simulink model "SIL_model"  (R2020a)
settings: Solver=ode4  StartTime=0.0  StopTime=30  FixedStep=0.001  RelTol=1e-3
InitFcn:
  | Init_control;
values from neighbouring files (symbols this model uses):
  layer1 = double(results{1,1}.layer9)    [load_parameter.m]
  layer2 = double(results{1,1}.layer10)    [load_parameter.m]
  layer3 = double(results{1,1}.layer11)    [load_parameter.m]
  layer4 = double(results{1,1}.layer12)    [load_parameter.m]
  layer5 = double(results{1,1}.layer13)    [load_parameter.m]
  layer6 = double(results{1,1}.layer14)    [load_parameter.m]
  std = sqrt(max(a,0.01))    [load_parameter.m]
undefined symbols (not defined in the file or in its folder): DWORK0, DWORK1, DWORK10, DWORK11, DWORK12, DWORK13, DWORK14, DWORK15, DWORK2, DWORK3, DWORK4, DWORK5, DWORK6, DWORK7, DWORK8, DWORK9, earthRadius, KiPitchAttitude, KiRollAttitude, Kp_RP_ANGLE, MAX_CONTROL_ANGLE_RATE_Y, MAX_CONTROL_ANGLE_RP, ModelInit_RPM, ModelParam_envAltitude, ModelParam_GlobalNoiseGainSwitch, ModelParam_GPSLatLong, ModelParam_motorCr, ModelParam_motorJm, ModelParam_motorMinThr, ModelParam_motorT, ModelParam_motorWb, ModelParam_rotorCm, ModelParam_rotorCt, ModelParam_uavCCm, ModelParam_uavCd, ModelParam_uavDearo, ModelParam_uavJ, ModelParam_uavMass, ModelParam_uavR, ModelParam_uavType, Receive, Send
libraries: aerolibfltsims x4, simulink x2, shared6dof x1, aerolibanimutils x1
(part 1 of 2)
settings Model: SimulationMode=accelerator  Creator=dream  LastModifiedBy=NEW
settings DataIOCC: ReturnWorkspaceOutputs=off
settings DebuggingCC: BusObjectLabelMismatch=error  ArithmeticOperatorsInVariantConditions=warning
settings SFSimCC: SimUseLocalCustomCode=off  CustomCodeUndefinedFunction=UseInterfaceOnly
settings RTWCC: RTWUseLocalCustomCode=off
settings CodeAppCC: StateflowObjectComments=on

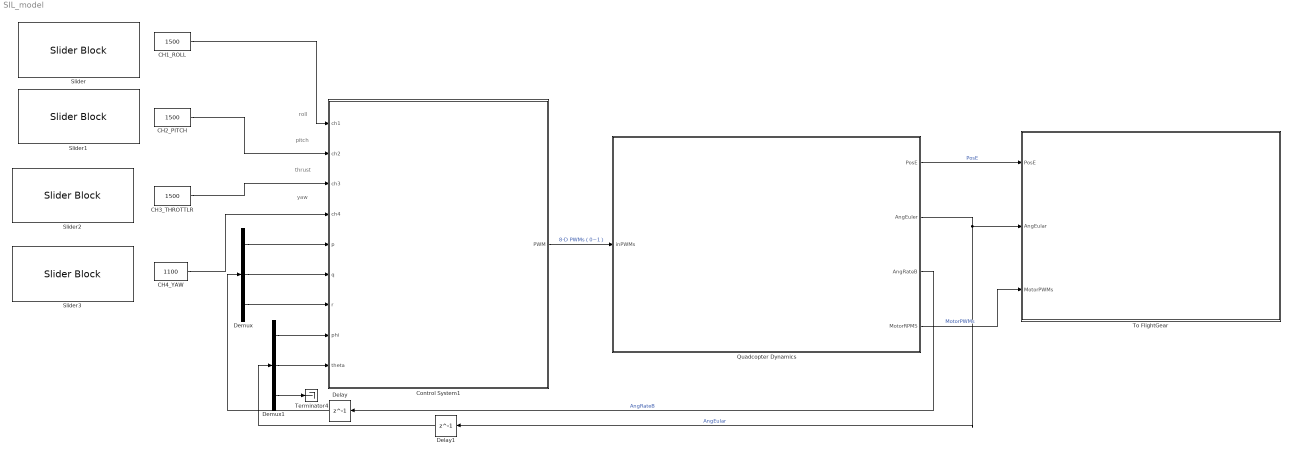
== system SIL_model ==
  note: roll
  note: pitch
  note: thrust
  note: yaw
  "     CH3_THROTTLR " : Constant  Value=1500  OutDataTypeStr=uint16
  "     CH4_YAW     " : Constant  Value=1100  OutDataTypeStr=uint16
  " CH2_PITCH " : Constant  Value=1500  OutDataTypeStr=uint16
  "CH1_ROLL   " : Constant  Value=1500  OutDataTypeStr=uint16
  Control System1 : Subsystem
      mask Display: image('icon\pixhawk.png');
  Delay : Delay  DelayLength=1  InitialCondition=0
  Delay1 : Delay  DelayLength=1  InitialCondition=0
  Demux : Demux  Outputs=3
  Demux1 : Demux  Outputs=3
  Quadcopter Dynamics : Subsystem
      mask Display: image('icon/F450.png');
  Slider : SliderBlock  ScaleMin=1100  ScaleMax=1900
  Slider1 : SliderBlock  ScaleMin=1100  ScaleMax=1900
  Slider2 : SliderBlock  ScaleMin=1500  ScaleMax=1680
  Slider3 : SliderBlock  ScaleMin=1100  ScaleMax=1900
  Terminator4 : Terminator
  To FlightGear : Subsystem
      mask Display: image('icon/FlightGear.png');
  wires:
  Quadcopter Dynamics/1(PosE) -> To FlightGear/1(PosE)  "PosE"
  Quadcopter Dynamics/2(AngEuler) -> To FlightGear/2(AngEular), Delay1/1  "AngEular"
  "CH1_ROLL   "/1 -> Control System1/1(ch1)
  "     CH4_YAW     "/1 -> Control System1/4(ch4)
  "     CH3_THROTTLR "/1 -> Control System1/3(ch3)
  Quadcopter Dynamics/3(AngRateB) -> Delay/1  "AngRateB"
  Demux/1 -> Control System1/5(p)
  Demux/2 -> Control System1/6(q)
  Demux/3 -> Control System1/7(r)
  Demux1/1 -> Control System1/8(phi)
  Demux1/2 -> Control System1/9(theta)
  Demux1/3 -> Terminator4/1
  " CH2_PITCH "/1 -> Control System1/2(ch2)
  Control System1/1(PWM) -> Quadcopter Dynamics/1(inPWMs)  "8-D PWMs（0~1）"
  Quadcopter Dynamics/4(MotorRPMS) -> To FlightGear/3(MotorPWMs)  "MotorPWMs"
  Delay/1 -> Demux/1
  Delay1/1 -> Demux1/1

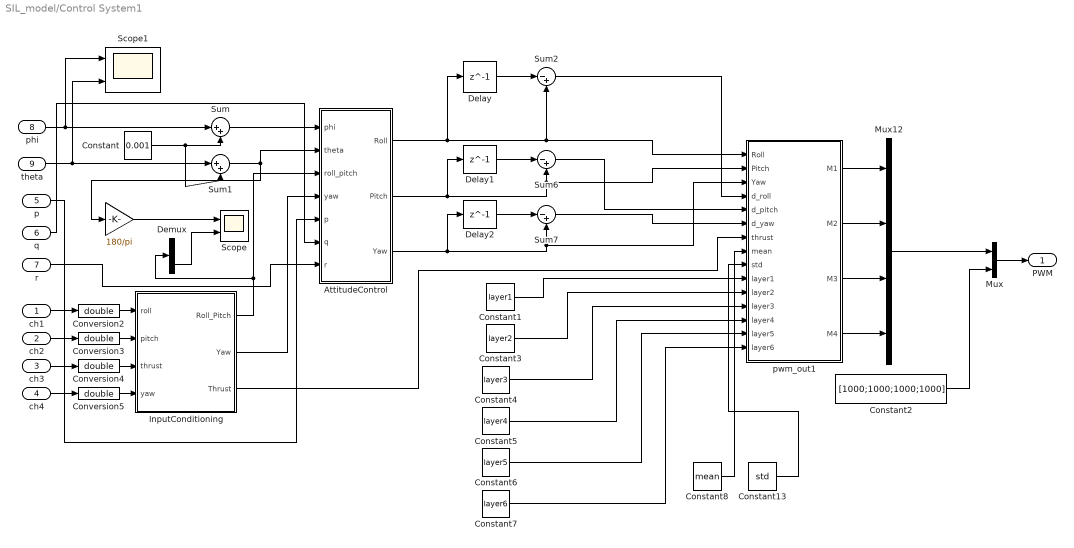
== system SIL_model/Control System1 ==
  ch1 : Inport  OutDataTypeStr=uint16  PortDimensions=1
  ch2 : Inport  Port=2  OutDataTypeStr=uint16  PortDimensions=1
  ch3 : Inport  Port=3  OutDataTypeStr=uint16  PortDimensions=1
  ch4 : Inport  Port=4  OutDataTypeStr=uint16  PortDimensions=1
  p : Inport  Port=5  PortDimensions=1
  q : Inport  Port=6  PortDimensions=1
  r : Inport  Port=7  PortDimensions=1
  phi : Inport  Port=8  PortDimensions=1
  theta : Inport  Port=9  PortDimensions=1
  " " : Gain  Gain=180/pi
  AttitudeControl : Subsystem
  Constant : Constant  Value=0.001
  Constant1 : Constant  Value=layer1
  Constant13 : Constant  Value=std
  Constant2 : Constant  Value=[1000;1000;1000;1000]
  Constant3 : Constant  Value=layer2
  Constant4 : Constant  Value=layer3
  Constant5 : Constant  Value=layer4
  Constant6 : Constant  Value=layer5
  Constant7 : Constant  Value=layer6
  Constant8 : Constant  Value=mean
  Conversion{2..5} (4 alike) : DataTypeConversion  OutDataTypeStr=double
  Delay : Delay  DelayLength=1  InitialCondition=0
  Delay1 : Delay  DelayLength=1  InitialCondition=0
  Delay2 : Delay  DelayLength=1  InitialCondition=0
  Demux : Demux  Outputs=2
  InputConditioning : Subsystem
  Mux : Mux  Inputs=2
  Mux12 : Mux
  Scope : Scope  NumInputPorts=2
  Scope1 : Scope  NumInputPorts=2
  Sum : Sum  Inputs=|++
  Sum1 : Sum  Inputs=|++
  Sum2 : Sum  Inputs=|-+
  Sum6 : Sum  Inputs=|-+
  Sum7 : Sum  Inputs=|-+
  pwm_out1 : MATLAB Function  TreatAsAtomicUnit=on
  PWM : Outport  PortDimensions=8  VectorParamsAs1DForOutWhenUnconnected=off
  wires:
  InputConditioning/3(Thrust) -> pwm_out1/7(thrust)
  AttitudeControl/2(Pitch) -> Delay1/1, Sum6/2, pwm_out1/2(Pitch)
  AttitudeControl/1(Roll) -> Delay/1, Sum2/2, pwm_out1/1(Roll)
  ch3/1 -> Conversion4/1
  pwm_out1/1(M1) -> Mux12/1
  pwm_out1/3(M3) -> Mux12/3
  pwm_out1/2(M2) -> Mux12/2
  r/1 -> AttitudeControl/7(r)
  AttitudeControl/3(Yaw) -> Delay2/1, Sum7/2, pwm_out1/3(Yaw)
  InputConditioning/1(Roll_Pitch) -> Demux/1, AttitudeControl/3(roll_pitch)
  q/1 -> AttitudeControl/6(q)
  theta/1 -> Scope1/2, Sum1/1
  InputConditioning/2(Yaw) -> AttitudeControl/4(yaw)
  p/1 -> AttitudeControl/5(p)
  ch4/1 -> Conversion5/1
  pwm_out1/4(M4) -> Mux12/4
  ch1/1 -> Conversion2/1
  ch2/1 -> Conversion3/1
  Conversion2/1 -> InputConditioning/1(roll)
  Conversion5/1 -> InputConditioning/4(yaw)
  Conversion4/1 -> InputConditioning/3(thrust)
  Conversion3/1 -> InputConditioning/2(pitch)
  " "/1 -> Scope/1
  Demux/2 -> Scope/2
  phi/1 -> Scope1/1, Sum/1
  Sum/1 -> AttitudeControl/1(phi)
  Sum1/1 -> " "/1, AttitudeControl/2(theta)
  Constant/1 -> Sum1/2, Sum/2
  Constant2/1 -> Mux/2
  Mux12/1 -> Mux/1
  Mux/1 -> PWM/1
  Sum2/1 -> pwm_out1/4(d_roll)
  Delay1/1 -> Sum6/1
  Sum6/1 -> pwm_out1/5(d_pitch)
  Delay2/1 -> Sum7/1
  Sum7/1 -> pwm_out1/6(d_yaw)
  Constant8/1 -> pwm_out1/8(mean)
  Constant13/1 -> pwm_out1/9(std)
  Constant1/1 -> pwm_out1/10(layer1)
  Constant3/1 -> pwm_out1/11(layer2)
  Constant4/1 -> pwm_out1/12(layer3)
  Constant5/1 -> pwm_out1/13(layer4)
  Constant6/1 -> pwm_out1/14(layer5)
  Constant7/1 -> pwm_out1/15(layer6)
  Delay/1 -> Sum2/1

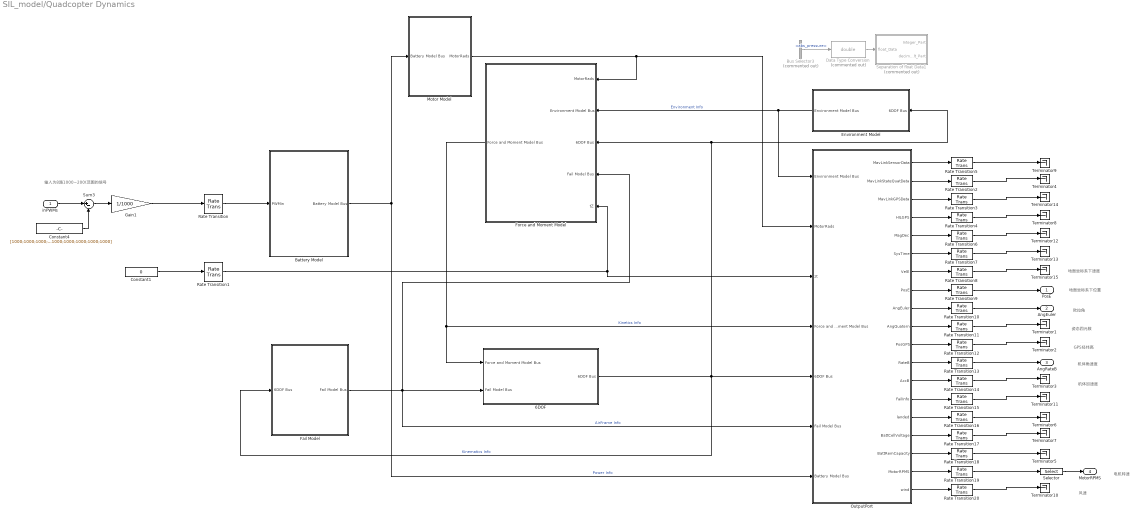
== system SIL_model/Quadcopter Dynamics ==
  note: 电机转速
  note: 风速
  note: 机体加速度
  note: 机体角速度
  note: GPS经纬高
  note: 姿态四元数
  note: 欧拉角
  note: 地面坐标系下位置
  note: 地面坐标系下速度
  note: 输入为8路1000~2000范围的信号
  inPWMs : Inport  PortDimensions=8
  6DOF : Subsystem
  Battery Model : Subsystem
      mask help: Simulink:masks:GenSFuncDesc_MD
      mask Help: eval('feval(''rtwprivate'',''rtwhelpview'',''rtw_sfcn_block'')');
  Bus Selector3 : BusSelector  Commented=on  OutputSignals=abs_pressure
  Constant1 : Constant  Value=0
  Constant4 : Constant  Value=[1000;1000;1000;1000;1000;1000;1000;1000]
  Data Type Conversion : DataTypeConversion  Commented=on  OutDataTypeStr=double
  Environment Model : Subsystem  mask{sfcnParam1=ModelParam_GPSLatLong, sfcnParam2=ModelParam_GlobalNoiseGainSwitch, sfcnParam3=ModelParam_envAltitude}
      mask prompts: sfcnParam1 "ModelParam_GPSLatLong:"; sfcnParam2 "ModelParam_GlobalNoiseGainSwitch:"; sfcnParam3 "ModelParam_envAltitude:"
      mask help: Simulink:masks:GenSFuncDesc_MD
      mask Help: eval('feval(''rtwprivate'',''rtwhelpview'',''rtw_sfcn_block'')');
  Fail Model : Subsystem  mask{sfcnParam1=ModelParam_uavJ, sfcnParam2=ModelParam_uavMass, sfcnParam3=ModelParam_uavR}
      mask prompts: sfcnParam1 "ModelParam_uavJ:"; sfcnParam2 "ModelParam_uavMass:"; sfcnParam3 "ModelParam_uavR:"
      mask help: Simulink:masks:GenSFuncDesc_MD
      mask Help: eval('feval(''rtwprivate'',''rtwhelpview'',''rtw_sfcn_block'')');
  Force and Moment Model : Subsystem  mask{sfcnParam1=ModelParam_motorJm, sfcnParam2=ModelParam_rotorCm, sfcnParam3=ModelParam_rotorCt, sfcnParam4=ModelParam_uavCCm, sfcnParam5=ModelParam_uavCd, sfcnParam6=ModelParam_uavDearo, sfcnParam7=ModelParam_uavR, sfcnParam8=ModelParam_uavType}
      mask prompts: sfcnParam1 "ModelParam_motorJm:"; sfcnParam2 "ModelParam_rotorCm:"; sfcnParam3 "ModelParam_rotorCt:"; sfcnParam4 "ModelParam_uavCCm:"; sfcnParam5 "ModelParam_uavCd:"; sfcnParam6 "ModelParam_uavDearo:"; sfcnParam7 "ModelParam_uavR:"; sfcnParam8 "ModelParam_uavType:"
      mask help: Simulink:masks:GenSFuncDesc_MD
      mask Help: eval('feval(''rtwprivate'',''rtwhelpview'',''rtw_sfcn_block'')');
  Gain1 : Gain  Gain=1/1000
  Motor Model : Subsystem  mask{sfcnParam1=ModelInit_RPM, sfcnParam2=ModelParam_motorCr, sfcnParam3=ModelParam_motorMinThr, sfcnParam4=ModelParam_motorT, sfcnParam5=ModelParam_motorWb}
      mask prompts: sfcnParam1 "ModelInit_RPM:"; sfcnParam2 "ModelParam_motorCr:"; sfcnParam3 "ModelParam_motorMinThr:"; sfcnParam4 "ModelParam_motorT:"; sfcnParam5 "ModelParam_motorWb:"
      mask help: Simulink:masks:GenSFuncDesc_MD
      mask Help: eval('feval(''rtwprivate'',''rtwhelpview'',''rtw_sfcn_block'')');
  OutputPort : Subsystem  mask{sfcnParam1=ModelParam_GPSLatLong, sfcnParam2=ModelParam_GlobalNoiseGainSwitch, sfcnParam3=ModelParam_envAltitude}
      mask prompts: sfcnParam1 "ModelParam_GPSLatLong:"; sfcnParam2 "ModelParam_GlobalNoiseGainSwitch:"; sfcnParam3 "ModelParam_envAltitude:"
      mask help: Simulink:masks:GenSFuncDesc_MD
      mask Help: eval('feval(''rtwprivate'',''rtwhelpview'',''rtw_sfcn_block'')');
  Rate Transition{,1..20} (21 alike) : RateTransition  OutPortSampleTime=ModelParam_BusSampleRate
  Selector : Selector  InputPortWidth=8  IndexOptions=Index vector (dialog)  Indices=[1 2 3 4]  OutputSizes=1
  Separation of float Data1 : Subsystem  Commented=on  mask{IntUint=1}
      mask prompts: IntUint "整数单位"
      mask help: 分离浮点数的整数和小数部分，这样在Labview MIT模块中可以稳定输出精度
  Sum3 : Sum  Inputs=|+-
  Terminator{1..15} (15 alike) : Terminator
  PosE : Outport  VectorParamsAs1DForOutWhenUnconnected=off
  AngEuler : Outport  Port=2  VectorParamsAs1DForOutWhenUnconnected=off
  AngRateB : Outport  Port=3  VectorParamsAs1DForOutWhenUnconnected=off
  MotorRPMS : Outport  Port=4  VectorParamsAs1DForOutWhenUnconnected=off
  wires:
  Selector/1 -> MotorRPMS/1
  Constant4/1 -> Sum3/2
  inPWMs/1 -> Sum3/1
  Constant1/1 -> Rate Transition1/1
  Sum3/1 -> Gain1/1
  Rate Transition5/1 -> Terminator9/1
  Rate Transition2/1 -> Terminator4/1
  Rate Transition3/1 -> Terminator14/1
  Rate Transition4/1 -> Terminator8/1
  Rate Transition6/1 -> Terminator12/1
  Rate Transition7/1 -> Terminator13/1
  Rate Transition8/1 -> Terminator15/1
  Rate Transition9/1 -> PosE/1
  Rate Transition10/1 -> AngEuler/1
  Rate Transition11/1 -> Terminator1/1
  Rate Transition12/1 -> Terminator2/1
  Rate Transition13/1 -> AngRateB/1
  Rate Transition14/1 -> Terminator3/1
  Rate Transition15/1 -> Terminator11/1
  Rate Transition16/1 -> Terminator6/1
  Rate Transition17/1 -> Terminator7/1
  Rate Transition18/1 -> Terminator5/1
  Rate Transition19/1 -> Selector/1
  Rate Transition20/1 -> Terminator10/1
  Gain1/1 -> Rate Transition/1
  OutputPort/2(MavLinkStateQuatData) -> Rate Transition2/1
  Motor Model/1(MotorRads) -> OutputPort/2(MotorRads), Force and Moment Model/1(MotorRads)
  OutputPort/15(landed) -> Rate Transition16/1
  OutputPort/3(MavLinkGPSData) -> Rate Transition3/1
  Bus Selector3/1 -> Data Type Conversion/1  "<abs_pressure>"
  Data Type Conversion/1 -> Separation of float Data1/1(float_Data)
  OutputPort/1(MavLinkSensorData) -> Rate Transition5/1
  OutputPort/14(FailInfo) -> Rate Transition15/1
  OutputPort/13(AccB) -> Rate Transition14/1
  OutputPort/12(RateB) -> Rate Transition13/1
  OutputPort/11(PosGPS) -> Rate Transition12/1
  OutputPort/10(AngQuatern) -> Rate Transition11/1
  OutputPort/9(AngEuler) -> Rate Transition10/1
  OutputPort/8(PosE) -> Rate Transition9/1
  OutputPort/7(VelE) -> Rate Transition8/1
  OutputPort/6(SysTime) -> Rate Transition7/1
  OutputPort/5(MagDec) -> Rate Transition6/1
  OutputPort/4(HILGPS) -> Rate Transition4/1
  Battery Model/1(Battery Model Bus) -> OutputPort/7(Battery Model Bus), Motor Model/1(Battery Model Bus)  "Power Info"
  Fail Model/1(Fail Model Bus) -> OutputPort/6(Fail Model Bus), Force and Moment Model/4(Fail Model Bus), 6DOF/2(Fail Model Bus)  "AirFrame Info"
  Force and Moment Model/1(Force and Moment Model Bus) -> OutputPort/4(Force and Moment Model Bus), 6DOF/1(Force and Moment Model Bus)  "Kinetics Info"
  6DOF/1(6DOF Bus) -> OutputPort/5(6DOF Bus), Fail Model/1(6DOF Bus), Environment Model/1(6DOF Bus), Force and Moment Model/3(6DOF Bus)  "Kinematics Info"
  Environment Model/1(Environment Model Bus) -> OutputPort/1(Environment Model Bus), Force and Moment Model/2(Environment Model Bus)  "Environment Info"
  OutputPort/16(BattCellVoltage) -> Rate Transition17/1
  OutputPort/17(BattRemCapacity) -> Rate Transition18/1
  OutputPort/19(wind) -> Rate Transition20/1
  OutputPort/18(MotorRPMS) -> Rate Transition19/1
  Rate Transition/1 -> Battery Model/1(PWMin)
  Rate Transition1/1 -> OutputPort/3(zt), Force and Moment Model/5("tZ ")

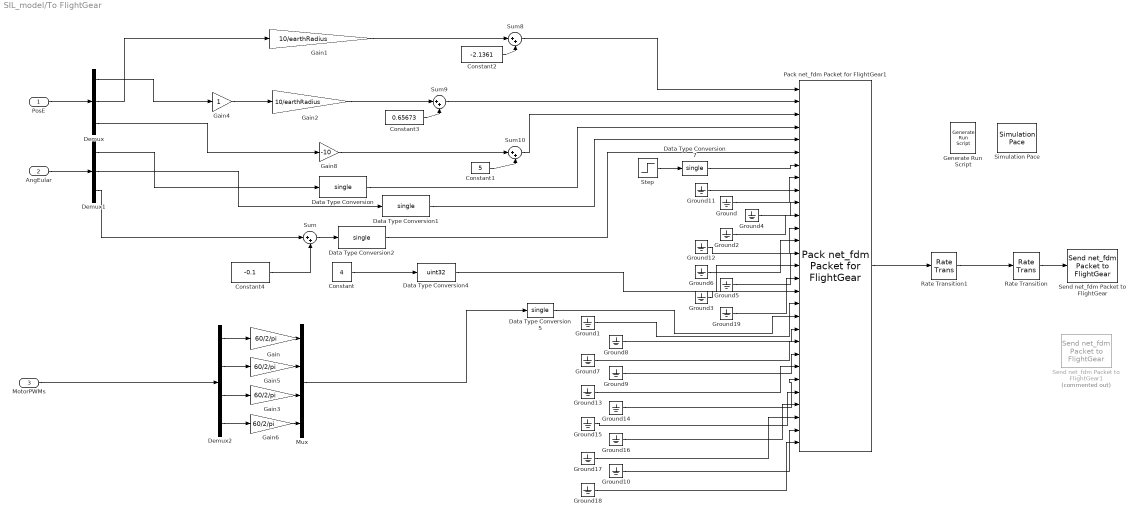
== system SIL_model/To FlightGear ==
  PosE : Inport
  AngEular : Inport  Port=2
  MotorPWMs : Inport  Port=3
  Constant : Constant  Value=4
  Constant1 : Constant  Value=5  VectorParams1D=off
  Constant2 : Constant  Value=-2.1361  VectorParams1D=off
  Constant3 : Constant  Value=0.65673  VectorParams1D=off
  Constant4 : Constant  Value=-0.1  VectorParams1D=off
  Data Type Conversion : DataTypeConversion  OutDataTypeStr=single  SaturateOnIntegerOverflow=on
  Data Type Conversion1 : DataTypeConversion  OutDataTypeStr=single  SaturateOnIntegerOverflow=on
  Data Type Conversion2 : DataTypeConversion  OutDataTypeStr=single  SaturateOnIntegerOverflow=on
  Data Type Conversion4 : DataTypeConversion  OutDataTypeStr=uint32
  Data Type Conversion5 : DataTypeConversion  OutDataTypeStr=single
  Data Type Conversion7 : DataTypeConversion  OutDataTypeStr=single
  Demux : Demux  Outputs=3
  Demux1 : Demux  Outputs=3
  Demux2 : Demux
  Gain{,3,5..6} (4 alike) : Gain  Gain=60/2/pi
  Gain1 : Gain  Gain=10/earthRadius
  Gain2 : Gain  Gain=10/earthRadius
  Gain4 : Gain
  Gain8 : Gain  Gain=-10
  Generate Run Script : aerolibfltsims/Generate Run Script  Architecture=Default  dataFlow=Send-Receive  GeometryModelName=Rotor4  AirportId=KSF0  RunwayId=10L  InitialAltitude=0  InitialHeading=0  OffsetDistance=0  OffsetAzimuth=0  InstallScenery=off  DisableShaders=off  OriginAddress=127.0.0.1  DestinationPort=5502  OriginPort=5505  LocalAddress=127.0.0.1  OutputFileName=runfg.bat  FlightGearBaseDirectory=C:\Program Files\FlightGear 2016.1.2
  Ground{,1..19} (20 alike) : Ground
  Mux : Mux
  Pack net_fdm Packet for FlightGear1 : aerolibfltsims/Pack net_fdm Packet for FlightGear  FlightGearVersion=v2016.1  ShowPositionAttitudeInputs=on  ShowVelocityAccelerationInputs=off  ShowControlSurfacePositionInputs=on  ShowEngineFuelInputs=on  ShowLandingGearInputs=off  ShowEnvironmentInputs=off  SampleTime=0.01  packetVersion=24
      settings: SourceProductBaseCode=AE
  Rate Transition : RateTransition
  Rate Transition1 : RateTransition
  Send net_fdm Packet to FlightGear : aerolibfltsims/Send net_fdm Packet to FlightGear  DestinationIpAddress=127.0.0.1  DestinationPort=5502  LocalIpPort=-1  varLen=off  SampleTime=0.005
      settings: SourceProductBaseCode=AE
  Send net_fdm Packet to FlightGear1 : aerolibfltsims/Send net_fdm Packet to FlightGear  Commented=on  DestinationIpAddress=192.168.199.46  DestinationPort=5502  LocalIpPort=-1  varLen=off  SampleTime=0.01
      settings: SourceProductBaseCode=AE
  Simulation Pace : aerolibanimutils/Simulation Pace  SimulationPace=1  SleepMode=MATLAB Thread  OutputPaceError=off  SampleTime=-1
      settings: AttributesFormatString=%<SimulationPace> sec/sec
  Step : Step  Time=5  SampleTime=0
  Sum{,8..10} (4 alike) : Sum  Inputs=|++
  wires:
  Rate Transition/1 -> Send net_fdm Packet to FlightGear/1
  Demux/1 -> Gain4/1
  Demux/2 -> Gain1/1
  Demux/3 -> Gain8/1
  Constant4/1 -> Sum/2
  Sum/1 -> Data Type Conversion2/1
  Gain1/1 -> Sum8/1
  Constant2/1 -> Sum8/2
  Gain2/1 -> Sum9/1
  Constant3/1 -> Sum9/2
  Constant1/1 -> Sum10/2
  Gain8/1 -> Sum10/1
  Pack net_fdm Packet for FlightGear1/1 -> Rate Transition1/1
  Demux1/2 -> Data Type Conversion1/1
  Demux1/3 -> Sum/1
  Data Type Conversion7/1 -> Pack net_fdm Packet for FlightGear1/7
  Ground8/1 -> Pack net_fdm Packet for FlightGear1/20
  Ground/1 -> Pack net_fdm Packet for FlightGear1/9
  Ground7/1 -> Pack net_fdm Packet for FlightGear1/21
  Ground9/1 -> Pack net_fdm Packet for FlightGear1/22
  Ground13/1 -> Pack net_fdm Packet for FlightGear1/23
  Ground14/1 -> Pack net_fdm Packet for FlightGear1/24
  Ground15/1 -> Pack net_fdm Packet for FlightGear1/25
  Ground16/1 -> Pack net_fdm Packet for FlightGear1/26
  Ground17/1 -> Pack net_fdm Packet for FlightGear1/27
  Ground10/1 -> Pack net_fdm Packet for FlightGear1/28
  Ground18/1 -> Pack net_fdm Packet for FlightGear1/29
  Step/1 -> Data Type Conversion7/1
  Data Type Conversion4/1 -> Pack net_fdm Packet for FlightGear1/17
  Ground1/1 -> Pack net_fdm Packet for FlightGear1/18
  Ground3/1 -> Pack net_fdm Packet for FlightGear1/15
  Ground5/1 -> Pack net_fdm Packet for FlightGear1/14
  Ground6/1 -> Pack net_fdm Packet for FlightGear1/13
  Ground4/1 -> Pack net_fdm Packet for FlightGear1/10
  Ground11/1 -> Pack net_fdm Packet for FlightGear1/8
  Data Type Conversion2/1 -> Pack net_fdm Packet for FlightGear1/6
  Data Type Conversion1/1 -> Pack net_fdm Packet for FlightGear1/5
  Data Type Conversion/1 -> Pack net_fdm Packet for FlightGear1/4
  Sum8/1 -> Pack net_fdm Packet for FlightGear1/1
  Sum9/1 -> Pack net_fdm Packet for FlightGear1/2
  Sum10/1 -> Pack net_fdm Packet for FlightGear1/3
  Constant/1 -> Data Type Conversion4/1
  Data Type Conversion5/1 -> Pack net_fdm Packet for FlightGear1/19
  Ground2/1 -> Pack net_fdm Packet for FlightGear1/11
  Ground12/1 -> Pack net_fdm Packet for FlightGear1/12
  Ground19/1 -> Pack net_fdm Packet for FlightGear1/16
  Gain4/1 -> Gain2/1
  AngEular/1 -> Demux1/1
  PosE/1 -> Demux/1
  MotorPWMs/1 -> Demux2/1
  Mux/1 -> Data Type Conversion5/1
  Demux2/1 -> Gain/1
  Demux2/3 -> Gain3/1
  Gain/1 -> Mux/1
  Gain3/1 -> Mux/3
  Demux2/2 -> Gain5/1
  Gain5/1 -> Mux/2
  Demux2/4 -> Gain6/1
  Gain6/1 -> Mux/4
  Demux1/1 -> Data Type Conversion/1
  Rate Transition1/1 -> Rate Transition/1

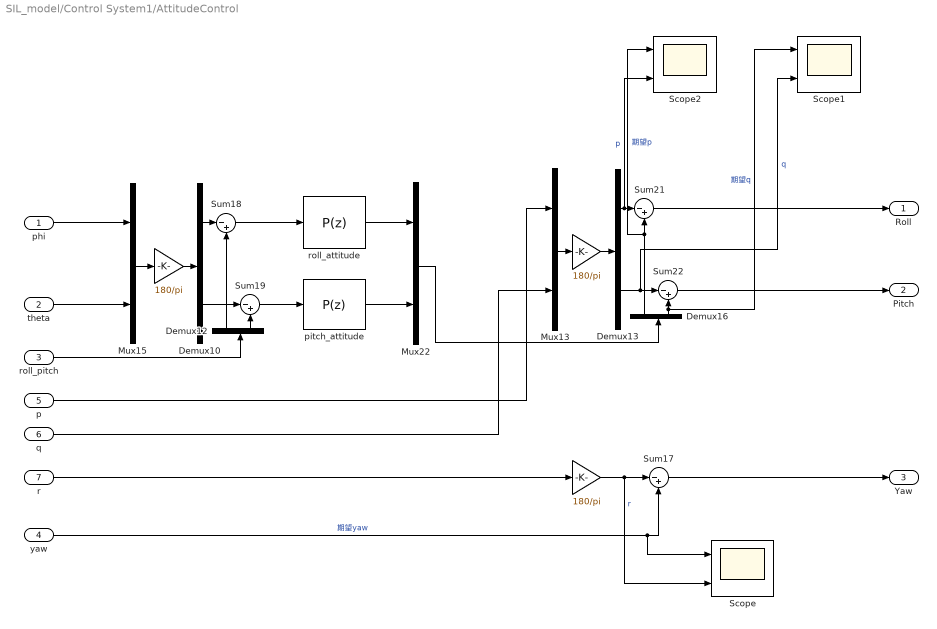
== system SIL_model/Control System1/AttitudeControl ==
  phi : Inport
  theta : Inport  Port=2
  roll_pitch : Inport  Port=3
  yaw : Inport  Port=4
  p : Inport  Port=5
  q : Inport  Port=6
  r : Inport  Port=7
  " " : Gain  Gain=180/pi
  "  " : Gain  Gain=180/pi
  "          " : Gain  Gain=180/pi
  Demux{10,12..13,16} (4 alike) : Demux  Outputs=2
  Mux13 : Mux  Inputs=2
  Mux15 : Mux  Inputs=2
  Mux22 : Mux  Inputs=2
  Scope : Scope  NumInputPorts=2
  Scope1 : Scope  NumInputPorts=2
  Scope2 : Scope  NumInputPorts=2
  Sum{17..19,21..22} (5 alike) : Sum  Inputs=|-+
  pitch_attitude : simulink/Continuous/PID Controller  Controller=P  Form=Parallel  TimeDomain=Discrete-time  UseExternalTs=off  SampleTime=-1  IntegratorMethod=Forward Euler  FilterMethod=Forward Euler  ControllerParametersSource=internal  P=Kp_RP_ANGLE  I=KiPitchAttitude  D=0.01  UseFilter=on  N=100  TunerSelectOption=Transfer Function Based (PID Tuner App)  InitialConditionSource=internal  InitialConditionForIntegrator=0  InitialConditionForFilter=0  DifferentiatorICPrevScaledInput=0  ExternalReset=none  TrackingMode=off  Kt=1  LimitOutput=on  UpperSaturationLimit=180  LowerSaturationLimit=-180  LinearizeAsGain=on  AntiWindupMode=back-calculation  Kb=1  POutMin=[]  POutMax=[]  IOutMin=[]  IOutMax=[]  DOutMin=[]  DOutMax=[]  NOutMin=[]  NOutMax=[]  SumOutMin=[]  SumOutMax=[]  SaturationOutMin=[]  SaturationOutMax=[]  PParamMin=[]  PParamMax=[]  IParamMin=[]  IParamMax=[]  DParamMin=[]  DParamMax=[]  NParamMin=[]  NParamMax=[]  KbParamMin=[]  KbParamMax=[]  KtParamMin=[]  KtParamMax=[]  KbOutMin=[]  KbOutMax=[]  KtOutMin=[]  KtOutMax=[]  IntegratorOutMin=[]  IntegratorOutMax=[]  FilterOutMin=[]  FilterOutMax=[]  SumI1OutMin=[]  SumI1OutMax=[]  SumI2OutMin=[]  SumI2OutMax=[]  SumI3OutMin=[]  SumI3OutMax=[]  SumI4OutMin=[]  SumI4OutMax=[]  SumDOutMin=[]  SumDOutMax=[]  DifferentiatorOutMin=[]  DifferentiatorOutMax=[]  FilterDiffOutCoefMin=[]  FilterDiffOutCoefMax=[]  ReciprocalOutMin=[]  ReciprocalOutMax=[]  SumDenOutMin=[]  SumDenOutMax=[]  SumNumOutMin=[]  SumNumOutMax=[]  DivideOutMin=[]  DivideOutMax=[]  UdiffTsProdOutMin=[]  UdiffTsProdOutMax=[]  NTsProdOutMin=[]  NTsProdOutMax=[]  UintegralTsProdOutMin=[]  UintegralTsProdOutMax=[]  UngainTsProdOutMin=[]  UngainTsProdOutMax=[]  IntegratorContinuousStateAttributes=''  IntegratorStateMustResolveToSignalObject=off  IntegratorRTWStateStorageClass=Auto  FilterContinuousStateAttributes=''  FilterStateMustResolveToSignalObject=off  FilterRTWStateStorageClass=Auto  ParallelPVariant=InternalParameters  IdealPVariant=Disabled  IVariant=Disabled  DVariant=Disabled  IntegratorVariant=Disabled  SatVariant=Enabled  AWVariant=Disabled  PCopyVariant=Disabled  TRVariant=Disabled  FdbkBlocksVariant=Forward  IdealPFdbkVariant=Disabled  SatFdbkVariant=Disabled  DerivativeFilterVariant=Disabled  NVariant=Disabled  NCopyVariant=Disabled_SignalSpec  FilterICVariant=Disabled  IntegratorICVariant=Disabled  ExternalResetVariant=Disabled  TRSumVariant=Passthrough  SumFdbkVariant=Disabled  SumVariant=Passthrough_P  TsampFilterVariant=InternalTs  TsampNgainVariant=Passthrough  TsampIntegralVariant=Disabled_SignalSpec
  roll_attitude : simulink/Continuous/PID Controller  Controller=P  Form=Parallel  TimeDomain=Discrete-time  UseExternalTs=off  SampleTime=-1  IntegratorMethod=Forward Euler  FilterMethod=Forward Euler  ControllerParametersSource=internal  P=Kp_RP_ANGLE  I=KiRollAttitude  D=0.01  UseFilter=on  N=100  TunerSelectOption=Transfer Function Based (PID Tuner App)  InitialConditionSource=internal  InitialConditionForIntegrator=0  InitialConditionForFilter=0  DifferentiatorICPrevScaledInput=0  ExternalReset=none  TrackingMode=off  Kt=1  LimitOutput=on  UpperSaturationLimit=180  LowerSaturationLimit=-180  LinearizeAsGain=on  AntiWindupMode=back-calculation  Kb=1  POutMin=[]  POutMax=[]  IOutMin=[]  IOutMax=[]  DOutMin=[]  DOutMax=[]  NOutMin=[]  NOutMax=[]  SumOutMin=[]  SumOutMax=[]  SaturationOutMin=[]  SaturationOutMax=[]  PParamMin=[]  PParamMax=[]  IParamMin=[]  IParamMax=[]  DParamMin=[]  DParamMax=[]  NParamMin=[]  NParamMax=[]  KbParamMin=[]  KbParamMax=[]  KtParamMin=[]  KtParamMax=[]  KbOutMin=[]  KbOutMax=[]  KtOutMin=[]  KtOutMax=[]  IntegratorOutMin=[]  IntegratorOutMax=[]  FilterOutMin=[]  FilterOutMax=[]  SumI1OutMin=[]  SumI1OutMax=[]  SumI2OutMin=[]  SumI2OutMax=[]  SumI3OutMin=[]  SumI3OutMax=[]  SumI4OutMin=[]  SumI4OutMax=[]  SumDOutMin=[]  SumDOutMax=[]  DifferentiatorOutMin=[]  DifferentiatorOutMax=[]  FilterDiffOutCoefMin=[]  FilterDiffOutCoefMax=[]  ReciprocalOutMin=[]  ReciprocalOutMax=[]  SumDenOutMin=[]  SumDenOutMax=[]  SumNumOutMin=[]  SumNumOutMax=[]  DivideOutMin=[]  DivideOutMax=[]  UdiffTsProdOutMin=[]  UdiffTsProdOutMax=[]  NTsProdOutMin=[]  NTsProdOutMax=[]  UintegralTsProdOutMin=[]  UintegralTsProdOutMax=[]  UngainTsProdOutMin=[]  UngainTsProdOutMax=[]  IntegratorContinuousStateAttributes=''  IntegratorStateMustResolveToSignalObject=off  IntegratorRTWStateStorageClass=Auto  FilterContinuousStateAttributes=''  FilterStateMustResolveToSignalObject=off  FilterRTWStateStorageClass=Auto  ParallelPVariant=InternalParameters  IdealPVariant=Disabled  IVariant=Disabled  DVariant=Disabled  IntegratorVariant=Disabled  SatVariant=Enabled  AWVariant=Disabled  PCopyVariant=Disabled  TRVariant=Disabled  FdbkBlocksVariant=Forward  IdealPFdbkVariant=Disabled  SatFdbkVariant=Disabled  DerivativeFilterVariant=Disabled  NVariant=Disabled  NCopyVariant=Disabled_SignalSpec  FilterICVariant=Disabled  IntegratorICVariant=Disabled  ExternalResetVariant=Disabled  TRSumVariant=Passthrough  SumFdbkVariant=Disabled  SumVariant=Passthrough_P  TsampFilterVariant=InternalTs  TsampNgainVariant=Passthrough  TsampIntegralVariant=Disabled_SignalSpec
  Roll : Outport  VectorParamsAs1DForOutWhenUnconnected=off
  Pitch : Outport  Port=2  VectorParamsAs1DForOutWhenUnconnected=off
  Yaw : Outport  Port=3  VectorParamsAs1DForOutWhenUnconnected=off
  wires:
  r/1 -> "          "/1
  q/1 -> Mux13/2
  Mux22/1 -> Demux16/1
  Sum17/1 -> Yaw/1
  phi/1 -> Mux15/1
  Mux15/1 -> " "/1
  theta/1 -> Mux15/2
  "          "/1 -> Scope/2, Sum17/1  "r"
  Sum19/1 -> pitch_attitude/1
  pitch_attitude/1 -> Mux22/2
  roll_attitude/1 -> Mux22/1
  Demux16/1 -> Scope2/1, Sum21/2  "期望p"
  yaw/1 -> Scope/1, Sum17/2  "期望yaw"
  roll_pitch/1 -> Demux12/1
  Demux16/2 -> Scope1/1, Sum22/2  "期望q"
  Demux12/1 -> Sum18/2
  Demux12/2 -> Sum19/2
  p/1 -> Mux13/1
  Demux10/1 -> Sum18/1
  Demux10/2 -> Sum19/1
  " "/1 -> Demux10/1
  Sum18/1 -> roll_attitude/1
  Sum22/1 -> Pitch/1
  Mux13/1 -> "  "/1
  Demux13/1 -> Scope2/2, Sum21/1  "p"
  Demux13/2 -> Scope1/2, Sum22/1  "q"
  "  "/1 -> Demux13/1
  Sum21/1 -> Roll/1

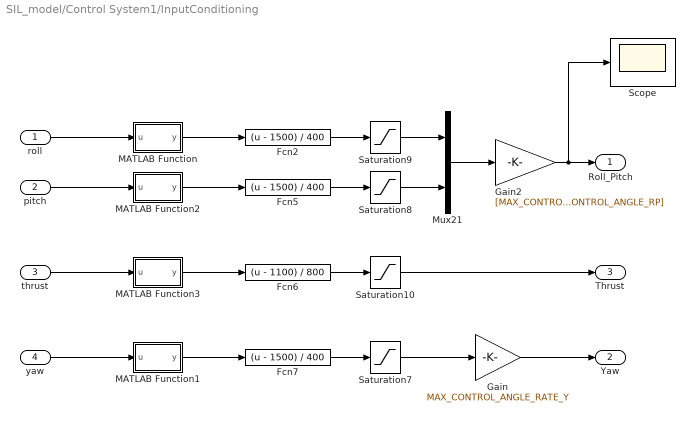
== system SIL_model/Control System1/InputConditioning ==
  roll : Inport
  pitch : Inport  Port=2
  thrust : Inport  Port=3
  yaw : Inport  Port=4
  Fcn2 : Fcn  Expr=(u - 1500) / 400
  Fcn5 : Fcn  Expr=(u - 1500) / 400
  Fcn6 : Fcn  Expr=(u - 1100) / 800
  Fcn7 : Fcn  Expr=(u - 1500) / 400
  Gain : Gain  Gain=MAX_CONTROL_ANGLE_RATE_Y
  Gain2 : Gain  Gain=[MAX_CONTROL_ANGLE_RP MAX_CONTROL_ANGLE_RP]  OutDataTypeStr=Inherit: Inherit via back propagation
  MATLAB Function : MATLAB Function  TreatAsAtomicUnit=on
  MATLAB Function1 : MATLAB Function  TreatAsAtomicUnit=on
  MATLAB Function2 : MATLAB Function  TreatAsAtomicUnit=on
  MATLAB Function3 : MATLAB Function  TreatAsAtomicUnit=on
  Mux21 : Mux  Inputs=2
  Saturation10 : Saturate  UpperLimit=1  LowerLimit=0
  Saturation7 : Saturate  UpperLimit=1  LowerLimit=-1
  Saturation8 : Saturate  UpperLimit=1  LowerLimit=-1
  Saturation9 : Saturate  UpperLimit=1  LowerLimit=-1
  Scope : Scope
  Roll_Pitch : Outport  VectorParamsAs1DForOutWhenUnconnected=off
  Yaw : Outport  Port=2  VectorParamsAs1DForOutWhenUnconnected=off
  Thrust : Outport  Port=3  VectorParamsAs1DForOutWhenUnconnected=off
  wires:
  Saturation10/1 -> Thrust/1
  Saturation7/1 -> Gain/1
  Gain2/1 -> Scope/1, Roll_Pitch/1
  Mux21/1 -> Gain2/1
  Saturation8/1 -> Mux21/2
  Fcn6/1 -> Saturation10/1
  Fcn2/1 -> Saturation9/1
  Fcn5/1 -> Saturation8/1
  Saturation9/1 -> Mux21/1
  Fcn7/1 -> Saturation7/1
  pitch/1 -> MATLAB Function2/1(u)
  MATLAB Function1/1(y) -> Fcn7/1
  thrust/1 -> MATLAB Function3/1(u)
  roll/1 -> MATLAB Function/1(u)
  MATLAB Function2/1(y) -> Fcn5/1
  MATLAB Function/1(y) -> Fcn2/1
  yaw/1 -> MATLAB Function1/1(u)
  MATLAB Function3/1(y) -> Fcn6/1
  Gain/1 -> Yaw/1

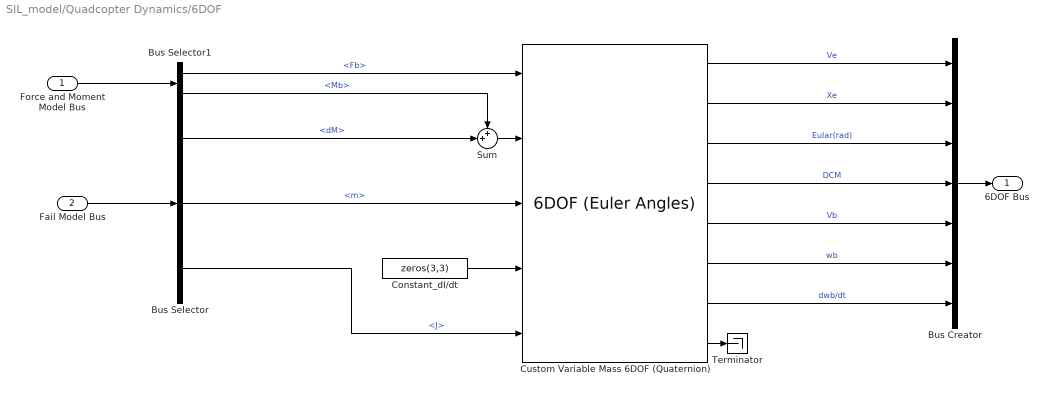
== system SIL_model/Quadcopter Dynamics/6DOF ==
  Force and Moment Model Bus : Inport
  Fail Model Bus : Inport  Port=2
  Bus Creator : BusCreator  Inputs=7
  Bus Selector : BusSelector  OutputSignals=dM,m,J
  Bus Selector1 : BusSelector  OutputSignals=Fb,Mb
  Constant_dI/dt : Constant  Value=zeros(3,3)
  Custom Variable Mass 6DOF (Quaternion) : shared6dof/6DOF (Euler Angles)  units=Metric (MKS)  mtype=Custom Variable  rep=Quaternion  xme_0=ModelInit_PosE  Vm_0=ModelInit_VelB  eul_0=ModelInit_AngEuler  pm_0=ModelInit_RateB  mass_0=1.0  mass_e=0.5  mass_f=2.0  inertia=eye(3)  inertia_e=eye(3)  inertia_f=2*eye(3)  k_quat=1.0  vre_flag=off  abi_flag=off  aMode=aMode  xme_statename=''  Vm_statename=''  eul_statename=''  quat_statename=''  pm_statename=''  mass_statename=''
      settings: SourceProductBaseCode=AE,PW,MT,VE,VP
  Sum : Sum  Inputs=++|
  Terminator : Terminator
  6DOF Bus : Outport  VectorParamsAs1DForOutWhenUnconnected=off
  wires:
  Bus Selector1/1 -> Custom Variable Mass 6DOF (Quaternion)/1  "<Fb>"
  Bus Selector/2 -> Custom Variable Mass 6DOF (Quaternion)/3  "<m>"
  Custom Variable Mass 6DOF (Quaternion)/8 -> Terminator/1
  Sum/1 -> Custom Variable Mass 6DOF (Quaternion)/2
  Constant_dI/dt/1 -> Custom Variable Mass 6DOF (Quaternion)/4
  Custom Variable Mass 6DOF (Quaternion)/5 -> Bus Creator/5  "Vb"
  Custom Variable Mass 6DOF (Quaternion)/6 -> Bus Creator/6  "wb"
  Custom Variable Mass 6DOF (Quaternion)/1 -> Bus Creator/1  "Ve"
  Custom Variable Mass 6DOF (Quaternion)/4 -> Bus Creator/4  "DCM"
  Custom Variable Mass 6DOF (Quaternion)/2 -> Bus Creator/2  "Xe"
  Custom Variable Mass 6DOF (Quaternion)/3 -> Bus Creator/3  "Eular(rad)"
  Custom Variable Mass 6DOF (Quaternion)/7 -> Bus Creator/7  "dwb/dt"
  Bus Selector/3 -> Custom Variable Mass 6DOF (Quaternion)/5  "<J>"
  Bus Selector/1 -> Sum/2  "<dM>"
  Bus Selector1/2 -> Sum/1  "<Mb>"
  Fail Model Bus/1 -> Bus Selector/1
  Force and Moment Model Bus/1 -> Bus Selector1/1
  Bus Creator/1 -> 6DOF Bus/1

== system SIL_model/Quadcopter Dynamics/Battery Model ==
  PWMin : Inport
  Battery Model_sfcn : S-Function  FunctionName=Battery_sf  SFunctionModules=""  SFunctionDeploymentMode=off  EnableBusSupport=off  mask{rtw_sf_name=Battery_sf, showVar=off}
      mask prompts: rtw_sf_name "Simulink:masks:GenSFuncName_MP"; showVar "Simulink:masks:GenSFuncShowModuleList_MP"
      mask help: Simulink:masks:GenSFuncDesc_MD
      mask init:
      | displist = '';
      | if ~strcmp(get_param(gcb, 'FunctionName'), rtw_sf_name);
      |   set_param(gcb, 'FunctionName', rtw_sf_name);
      | end
      | % Check if we are generating code
      | rtw_mode = false;
      | if strcmpi(get_param(bdroot(gcb),'SimulationStatus'),'Initializing')
      | 	rtw_mode = strcmpi(get_param(bdroot(gcb),'BuildingRTWCode'),'on') && ...
      | 		~strcmpi(get_param(bdroot(gcb),'TargetStyle'),'SimulationTarget');
      | end
      | if showVar || rtw_mode
      | 	if exist('rtwsfunc') == 2 | exist('rtwsfunc') == 6
      | 		tmplist = rtwsfunc(rtw_sf_name,gcb);
      | 		tmplist = DAStudio.message('Simulink:masks:GenSFuncListOfModules_IC', tmplist);
      | 	elseif showVar
      | 		tmplist1 = DAStudio.message('Simulink:masks:GenSFuncListOfModules_IC', '');
      |         tmplist2 = DAStudio.message('Simulink:masks:GenSFuncNotLicensed_IC');
      |         tmplist = [tmplist1 tmplist2];
      |  	end
      | end
      | if showVar
      |   displist = tmplist;
      | end
      settings: CopyFcn=|
      | if ~strcmp(get_param(gcb,'Linkstatus'),'none') && ...
      | ~strcmp(get_param(gcb,'Linkstatus'),'implicit')
      |   set_param(gcb,'LinkStatus','none');
      | end
      mask Help: eval('feval(''rtwprivate'',''rtwhelpview'',''rtw_sfcn_block'')');
      mask Display:
      | port_label('input',1,'PWMin');
      | port_label('output',1,'PWMOut');
      | port_label('output',2,'cellVol');
      | port_label('output',3,'remCapa');
  __InputSSForSFun__ : Subsystem
  __OutputSSForSFun__ : Subsystem
  Battery Model Bus : Outport  VectorParamsAs1DForOutWhenUnconnected=off
  wires:
  PWMin/1 -> __InputSSForSFun__/1(PWMin)
  __InputSSForSFun__/1(__UniqueOutportName__1__) -> Battery Model_sfcn/1
  Battery Model_sfcn/1 -> __OutputSSForSFun__/1(__UniqueInportName__1__)
  Battery Model_sfcn/2 -> __OutputSSForSFun__/2(__UniqueInportName__2__)
  Battery Model_sfcn/3 -> __OutputSSForSFun__/3(__UniqueInportName__3__)
  __OutputSSForSFun__/1(Battery Model Bus) -> Battery Model Bus/1

== system SIL_model/Quadcopter Dynamics/Environment Model ==
  6DOF Bus : Inport
  Environment Model_sfcn : S-Function  FunctionName=Environment_sf  Parameters=sfcnParam1, sfcnParam2, sfcnParam3  SFunctionModules=""  SFunctionDeploymentMode=off  EnableBusSupport=off  SFcnStateName=DWORK0,DWORK1,DWORK2,DWORK3,DWORK4,DWORK5,DWORK6,DWORK7,DWORK8,DWORK9,DWORK10,DWORK11,DWORK12,DWORK13,DWORK14,DWORK15  mask{rtw_sf_name=Environment_sf, showVar=off, sfcnParam1=sfcnParam1, sfcnParam2=sfcnParam2, sfcnParam3=sfcnParam3}
      mask prompts: rtw_sf_name "Simulink:masks:GenSFuncName_MP"; showVar "Simulink:masks:GenSFuncShowModuleList_MP"; sfcnParam1 "ModelParam_GPSLatLong:"; sfcnParam2 "ModelParam_GlobalNoiseGainSwitch:"; sfcnParam3 "ModelParam_envAltitude:"
      mask help: Simulink:masks:GenSFuncDesc_MD
      mask init: same as SIL_model/Quadcopter Dynamics/Battery Model/Battery Model_sfcn
      settings: SFcnIsStateOwnerBlock=on
      settings: CopyFcn=|
      | if ~strcmp(get_param(gcb,'Linkstatus'),'none') && ...
      | ~strcmp(get_param(gcb,'Linkstatus'),'implicit')
      |   set_param(gcb,'LinkStatus','none');
      | end
      mask Help: eval('feval(''rtwprivate'',''rtwhelpview'',''rtw_sfcn_block'')');
      mask Display:
      | port_label('input',1,'Ve');
      | port_label('input',2,'Xe');
      | port_label('input',3,'Eular(rad)');
      | port_label('input',4,'DCM');
      | port_label('input',5,'Vb');
      | port_label('input',6,'wb');
      | port_label('input',7,'dwb/dt');
      | port_label('output',1,'PosGPS');
      | port_label('output',2,'gravity');
      | port_label('output',3,'TempC');
      | port_label('output',4,'AirPressure');
      | port_label('output',5,'Rho');
      | port_label('output',6,'Windb');
      | port_label('output',7,'Wind');
  __InputSSForSFun__ : Subsystem
  __OutputSSForSFun__ : Subsystem
  Environment Model Bus : Outport  VectorParamsAs1DForOutWhenUnconnected=off
  wires:
  6DOF Bus/1 -> __InputSSForSFun__/1(6DOF Bus)
  __InputSSForSFun__/1(__UniqueOutportName__1__) -> Environment Model_sfcn/1
  __InputSSForSFun__/2(__UniqueOutportName__2__) -> Environment Model_sfcn/2
  __InputSSForSFun__/3(__UniqueOutportName__3__) -> Environment Model_sfcn/3
  __InputSSForSFun__/4(__UniqueOutportName__4__) -> Environment Model_sfcn/4
  __InputSSForSFun__/5(__UniqueOutportName__5__) -> Environment Model_sfcn/5
  __InputSSForSFun__/6(__UniqueOutportName__6__) -> Environment Model_sfcn/6
  __InputSSForSFun__/7(__UniqueOutportName__7__) -> Environment Model_sfcn/7
  Environment Model_sfcn/1 -> __OutputSSForSFun__/1(__UniqueInportName__1__)
  Environment Model_sfcn/2 -> __OutputSSForSFun__/2(__UniqueInportName__2__)
  Environment Model_sfcn/3 -> __OutputSSForSFun__/3(__UniqueInportName__3__)
  Environment Model_sfcn/4 -> __OutputSSForSFun__/4(__UniqueInportName__4__)
  Environment Model_sfcn/5 -> __OutputSSForSFun__/5(__UniqueInportName__5__)
  Environment Model_sfcn/6 -> __OutputSSForSFun__/6(__UniqueInportName__6__)
  Environment Model_sfcn/7 -> __OutputSSForSFun__/7(__UniqueInportName__7__)
  __OutputSSForSFun__/1(Environment Model Bus) -> Environment Model Bus/1

== system SIL_model/Quadcopter Dynamics/Fail Model ==
  6DOF Bus : Inport
  Fail Model_sfcn : S-Function  FunctionName=Fail_sf  Parameters=sfcnParam1, sfcnParam2, sfcnParam3  SFunctionModules=""  SFunctionDeploymentMode=off  EnableBusSupport=off  mask{rtw_sf_name=Fail_sf, showVar=off, sfcnParam1=sfcnParam1, sfcnParam2=sfcnParam2, sfcnParam3=sfcnParam3}
      mask prompts: rtw_sf_name "Simulink:masks:GenSFuncName_MP"; showVar "Simulink:masks:GenSFuncShowModuleList_MP"; sfcnParam1 "ModelParam_uavJ:"; sfcnParam2 "ModelParam_uavMass:"; sfcnParam3 "ModelParam_uavR:"
      mask help: Simulink:masks:GenSFuncDesc_MD
      mask init: same as SIL_model/Quadcopter Dynamics/Battery Model/Battery Model_sfcn
      settings: CopyFcn=|
      | if ~strcmp(get_param(gcb,'Linkstatus'),'none') && ...
      | ~strcmp(get_param(gcb,'Linkstatus'),'implicit')
      |   set_param(gcb,'LinkStatus','none');
      | end
      mask Help: eval('feval(''rtwprivate'',''rtwhelpview'',''rtw_sfcn_block'')');
      mask Display:
      | port_label('input',1,'Ve');
      | port_label('input',2,'Xe');
      | port_label('input',3,'Eular(rad)');
      | port_label('input',4,'DCM');
      | port_label('input',5,'Vb');
      | port_label('input',6,'wb');
      | port_label('input',7,'dwb/dt');
      | port_label('output',1,'m');
      | port_label('output',2,'J');
      | port_label('output',3,'dM');
  __InputSSForSFun__ : Subsystem
  __OutputSSForSFun__ : Subsystem
  Fail Model Bus : Outport  VectorParamsAs1DForOutWhenUnconnected=off
  wires:
  6DOF Bus/1 -> __InputSSForSFun__/1(6DOF Bus)
  __InputSSForSFun__/1(__UniqueOutportName__1__) -> Fail Model_sfcn/1
  __InputSSForSFun__/2(__UniqueOutportName__2__) -> Fail Model_sfcn/2
  __InputSSForSFun__/3(__UniqueOutportName__3__) -> Fail Model_sfcn/3
  __InputSSForSFun__/4(__UniqueOutportName__4__) -> Fail Model_sfcn/4
  __InputSSForSFun__/5(__UniqueOutportName__5__) -> Fail Model_sfcn/5
  __InputSSForSFun__/6(__UniqueOutportName__6__) -> Fail Model_sfcn/6
  __InputSSForSFun__/7(__UniqueOutportName__7__) -> Fail Model_sfcn/7
  Fail Model_sfcn/1 -> __OutputSSForSFun__/1(__UniqueInportName__1__)
  Fail Model_sfcn/2 -> __OutputSSForSFun__/2(__UniqueInportName__2__)
  Fail Model_sfcn/3 -> __OutputSSForSFun__/3(__UniqueInportName__3__)
  __OutputSSForSFun__/1(Fail Model Bus) -> Fail Model Bus/1

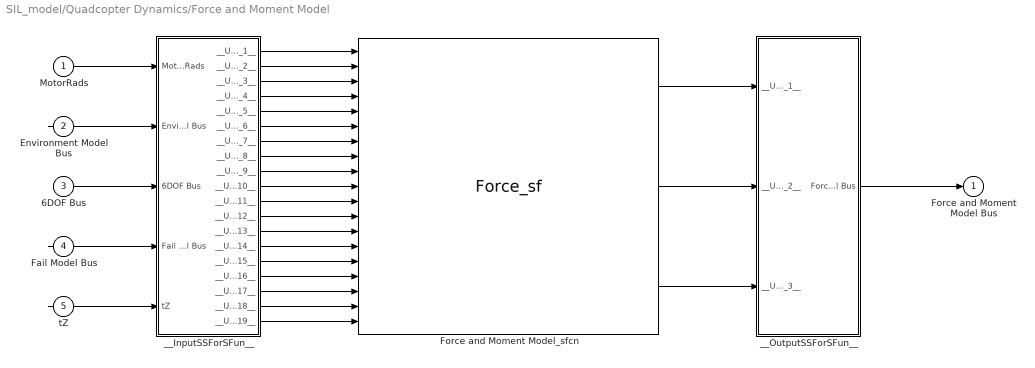
== system SIL_model/Quadcopter Dynamics/Force and Moment Model ==
  MotorRads : Inport
  Environment Model Bus : Inport  Port=2
  6DOF Bus : Inport  Port=3
  Fail Model Bus : Inport  Port=4
  "tZ " : Inport  Port=5
  Force and Moment Model_sfcn : S-Function  FunctionName=Force_sf  Parameters=sfcnParam1, sfcnParam2, sfcnParam3, sfcnParam4, sfcnParam5, sfcnParam6, sfcnParam7, sfcnParam8  SFunctionModules=""  SFunctionDeploymentMode=off  EnableBusSupport=off  mask{rtw_sf_name=Force_sf, showVar=off, sfcnParam1=sfcnParam1, sfcnParam2=sfcnParam2, sfcnParam3=sfcnParam3, sfcnParam4=sfcnParam4, sfcnParam5=sfcnParam5, sfcnParam6=sfcnParam6, sfcnParam7=sfcnParam7, sfcnParam8=sfcnParam8}
      mask prompts: rtw_sf_name "Simulink:masks:GenSFuncName_MP"; showVar "Simulink:masks:GenSFuncShowModuleList_MP"; sfcnParam1 "ModelParam_motorJm:"; sfcnParam2 "ModelParam_rotorCm:"; sfcnParam3 "ModelParam_rotorCt:"; sfcnParam4 "ModelParam_uavCCm:"; sfcnParam5 "ModelParam_uavCd:"; sfcnParam6 "ModelParam_uavDearo:"; sfcnParam7 "ModelParam_uavR:"; sfcnParam8 "ModelParam_uavType:"
      mask help: Simulink:masks:GenSFuncDesc_MD
      mask init: same as SIL_model/Quadcopter Dynamics/Battery Model/Battery Model_sfcn
      settings: CopyFcn=|
      | if ~strcmp(get_param(gcb,'Linkstatus'),'none') && ...
      | ~strcmp(get_param(gcb,'Linkstatus'),'implicit')
      |   set_param(gcb,'LinkStatus','none');
      | end
      mask Help: eval('feval(''rtwprivate'',''rtwhelpview'',''rtw_sfcn_block'')');
      mask Display:
      | port_label('input',1,'MotorRads');
      | port_label('input',2,'PosGPS');
      | port_label('input',3,'gravity');
      | port_label('input',4,'TempC');
      | port_label('input',5,'AirPressure');
      | port_label('input',6,'Rho');
      | port_label('input',7,'Windb');
      | port_label('input',8,'Wind');
      | port_label('input',9,'Ve');
      | port_label('input',10,'Xe');
      | port_label('input',11,'Eular(rad)');
      | port_label('input',12,'DCM');
      | port_label('input',13,'Vb');
      | port_label('input',14,'wb');
      | port_label('input',15,'dwb/dt');
      | port_label('input',16,'m');
      | port_label('input',17,'J');
      | port_label('input',18,'dM');
      | port_label('input',19,'tZ ');
      | port_label('output',1,'Fb');
      | port_label('output',2,'Mb');
      | port_label('output',3,'landed');
  __InputSSForSFun__ : Subsystem
  __OutputSSForSFun__ : Subsystem
  Force and Moment Model Bus : Outport  VectorParamsAs1DForOutWhenUnconnected=off
  wires:
  MotorRads/1 -> __InputSSForSFun__/1(MotorRads)
  Environment Model Bus/1 -> __InputSSForSFun__/2(Environment Model Bus)
  6DOF Bus/1 -> __InputSSForSFun__/3(6DOF Bus)
  Fail Model Bus/1 -> __InputSSForSFun__/4(Fail Model Bus)
  "tZ "/1 -> __InputSSForSFun__/5("tZ ")
  __InputSSForSFun__/1(__UniqueOutportName__1__) -> Force and Moment Model_sfcn/1
  __InputSSForSFun__/2(__UniqueOutportName__2__) -> Force and Moment Model_sfcn/2
  __InputSSForSFun__/3(__UniqueOutportName__3__) -> Force and Moment Model_sfcn/3
  __InputSSForSFun__/4(__UniqueOutportName__4__) -> Force and Moment Model_sfcn/4
  __InputSSForSFun__/5(__UniqueOutportName__5__) -> Force and Moment Model_sfcn/5
  __InputSSForSFun__/6(__UniqueOutportName__6__) -> Force and Moment Model_sfcn/6
  __InputSSForSFun__/7(__UniqueOutportName__7__) -> Force and Moment Model_sfcn/7
  __InputSSForSFun__/8(__UniqueOutportName__8__) -> Force and Moment Model_sfcn/8
  __InputSSForSFun__/9(__UniqueOutportName__9__) -> Force and Moment Model_sfcn/9
  __InputSSForSFun__/10(__UniqueOutportName__10__) -> Force and Moment Model_sfcn/10
  __InputSSForSFun__/11(__UniqueOutportName__11__) -> Force and Moment Model_sfcn/11
  __InputSSForSFun__/12(__UniqueOutportName__12__) -> Force and Moment Model_sfcn/12
  __InputSSForSFun__/13(__UniqueOutportName__13__) -> Force and Moment Model_sfcn/13
  __InputSSForSFun__/14(__UniqueOutportName__14__) -> Force and Moment Model_sfcn/14
  __InputSSForSFun__/15(__UniqueOutportName__15__) -> Force and Moment Model_sfcn/15
  __InputSSForSFun__/16(__UniqueOutportName__16__) -> Force and Moment Model_sfcn/16
  __InputSSForSFun__/17(__UniqueOutportName__17__) -> Force and Moment Model_sfcn/17
  __InputSSForSFun__/18(__UniqueOutportName__18__) -> Force and Moment Model_sfcn/18
  __InputSSForSFun__/19(__UniqueOutportName__19__) -> Force and Moment Model_sfcn/19
  Force and Moment Model_sfcn/1 -> __OutputSSForSFun__/1(__UniqueInportName__1__)
  Force and Moment Model_sfcn/2 -> __OutputSSForSFun__/2(__UniqueInportName__2__)
  Force and Moment Model_sfcn/3 -> __OutputSSForSFun__/3(__UniqueInportName__3__)
  __OutputSSForSFun__/1(Force and Moment Model Bus) -> Force and Moment Model Bus/1

== system SIL_model/Quadcopter Dynamics/Motor Model ==
  Battery Model Bus : Inport
  Motor Model_sfcn : S-Function  FunctionName=Motor_sf  Parameters=sfcnParam1, sfcnParam2, sfcnParam3, sfcnParam4, sfcnParam5  SFunctionModules=""  SFunctionDeploymentMode=off  EnableBusSupport=off  mask{rtw_sf_name=Motor_sf, showVar=off, sfcnParam1=sfcnParam1, sfcnParam2=sfcnParam2, sfcnParam3=sfcnParam3, sfcnParam4=sfcnParam4, sfcnParam5=sfcnParam5}
      mask prompts: rtw_sf_name "Simulink:masks:GenSFuncName_MP"; showVar "Simulink:masks:GenSFuncShowModuleList_MP"; sfcnParam1 "ModelInit_RPM:"; sfcnParam2 "ModelParam_motorCr:"; sfcnParam3 "ModelParam_motorMinThr:"; sfcnParam4 "ModelParam_motorT:"; sfcnParam5 "ModelParam_motorWb:"
      mask help: Simulink:masks:GenSFuncDesc_MD
      mask init: same as SIL_model/Quadcopter Dynamics/Battery Model/Battery Model_sfcn
      settings: CopyFcn=|
      | if ~strcmp(get_param(gcb,'Linkstatus'),'none') && ...
      | ~strcmp(get_param(gcb,'Linkstatus'),'implicit')
      |   set_param(gcb,'LinkStatus','none');
      | end
      mask Help: eval('feval(''rtwprivate'',''rtwhelpview'',''rtw_sfcn_block'')');
      mask Display:
      | port_label('input',1,'PWMOut');
      | port_label('input',2,'cellVol');
      | port_label('input',3,'remCapa');
      | port_label('output',1,'MotorRads');
  __InputSSForSFun__ : Subsystem
  __OutputSSForSFun__ : Subsystem
  MotorRads : Outport  VectorParamsAs1DForOutWhenUnconnected=off
  wires:
  Battery Model Bus/1 -> __InputSSForSFun__/1(Battery Model Bus)
  __InputSSForSFun__/1(__UniqueOutportName__1__) -> Motor Model_sfcn/1
  __InputSSForSFun__/2(__UniqueOutportName__2__) -> Motor Model_sfcn/2
  __InputSSForSFun__/3(__UniqueOutportName__3__) -> Motor Model_sfcn/3
  Motor Model_sfcn/1 -> __OutputSSForSFun__/1(__UniqueInportName__1__)
  __OutputSSForSFun__/1(MotorRads) -> MotorRads/1
